simulink library "induction_machine"  (R2025b)
settings: Solver=VariableStepAuto  StartTime=0.0  StopTime=10.0  RelTol=1e-3
undefined symbols (not defined in the file): cp, Jm_model, Lm, Lr, Ls, Rr, Rs
libraries: nesl_utility x41, fl_lib x1, im_uvw_2_lib x1
settings Model: Creator=dbagn  LastModifiedBy=ltnbda

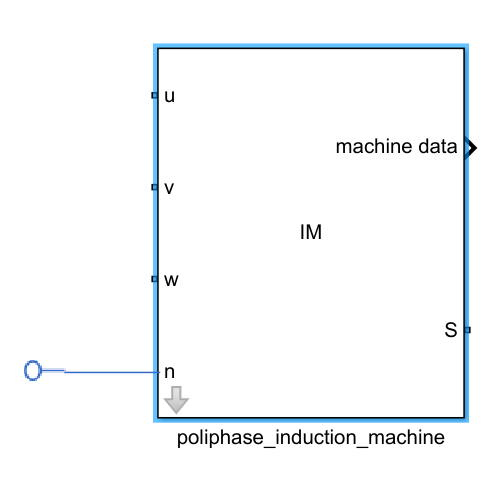
[thumbnail: Simulink's stored preview of the top-level diagram]
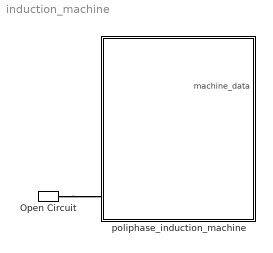
== system induction_machine ==
  Open Circuit : fl_lib/Electrical/Electrical Elements/Open Circuit  v_specify=off  v_priority=None  v=0 V  v_nominal_specify=off  v_nominal_value=1  v_nominal_unit=V
  poliphase_induction_machine : Subsystem  mask{Rs_m=Rs, Ls_m=Ls, Lm_m=Lm, Lr_m=Lr, Rr_m=Rr, Jm_m=Jm_model, bm_m=Tn/omega_m_nom/3, cp_m=cp}
      mask prompts: Rs_m "Stator resistance - Rs [Ohm]"; Ls_m "Stator inductance - Ls [H]"; Lm_m "Mutual inductance - Lm [H]"; Lr_m "Rotor inductance - Lr [H]"; Rr_m "Rotor resistance - Rr [Ohm]"; Jm_m "Load inertia - Jm [kgm^2]"; bm_m "Loadviscosity - bm [Nm*s/rad]"; cp_m "Number of pole pairs"
      mask Display:
      | disp('IM');
      | port_label('lconn', 1, 'u');
      | port_label('lconn', 2, 'v');
      | port_label('lconn', 3, 'w');
      | port_label('lconn', 4, 'n');
      | port_label('output', 1, 'machine data');
      | port_label('rconn',1, 'S');
  connections:
  Open Circuit/LConn1 -- poliphase_induction_machine/LConn4

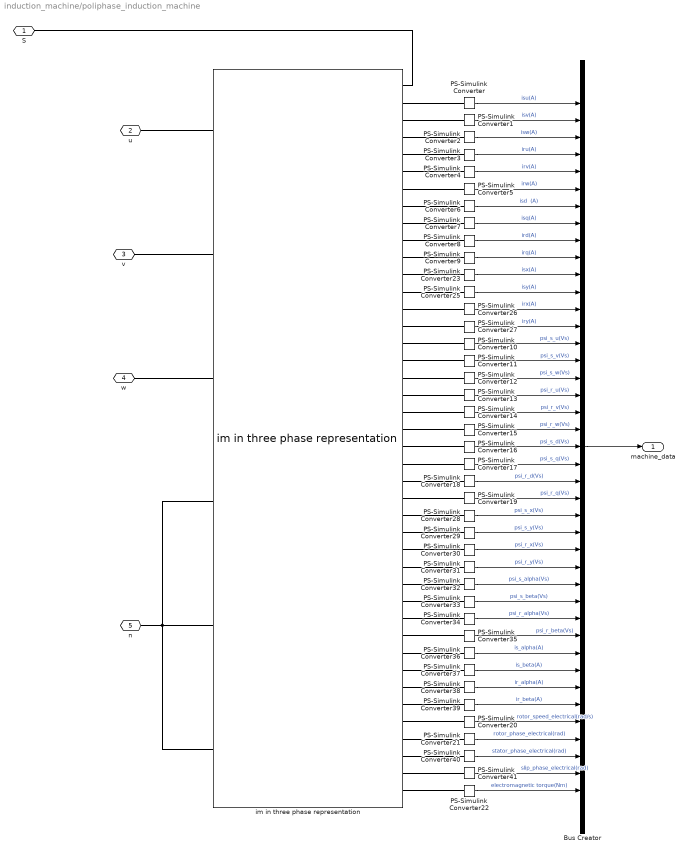
== system induction_machine/poliphase_induction_machine ==
  Bus Creator : BusCreator  Inputs=41
  PS-Simulink Converter{,1..9,23,25..27,36..39} (18 alike) : nesl_utility/PS-Simulink Converter  PhysicalDomain=network_engine_domain  SubClassName=ps_output  LeftPortType=input  RightPortType=output  PseudoPeriodic=off  Frequencies=[]  VectorFormat=1-D array  Unit=A  AffineConversion=off
  PS-Simulink Converter{10..19,28..35} (18 alike) : nesl_utility/PS-Simulink Converter  PhysicalDomain=network_engine_domain  SubClassName=ps_output  LeftPortType=input  RightPortType=output  PseudoPeriodic=off  Frequencies=[]  VectorFormat=1-D array  Unit=V*s  AffineConversion=off
  PS-Simulink Converter20 : nesl_utility/PS-Simulink Converter  PhysicalDomain=network_engine_domain  SubClassName=ps_output  LeftPortType=input  RightPortType=output  PseudoPeriodic=off  Frequencies=[]  VectorFormat=1-D array  Unit=rad/s  AffineConversion=off
  PS-Simulink Converter21 : nesl_utility/PS-Simulink Converter  PhysicalDomain=network_engine_domain  SubClassName=ps_output  LeftPortType=input  RightPortType=output  PseudoPeriodic=off  Frequencies=[]  VectorFormat=1-D array  Unit=rad  AffineConversion=off
  PS-Simulink Converter22 : nesl_utility/PS-Simulink Converter  PhysicalDomain=network_engine_domain  SubClassName=ps_output  LeftPortType=input  RightPortType=output  PseudoPeriodic=off  Frequencies=[]  VectorFormat=1-D array  Unit=N*m  AffineConversion=off
  PS-Simulink Converter40 : nesl_utility/PS-Simulink Converter  PhysicalDomain=network_engine_domain  SubClassName=ps_output  LeftPortType=input  RightPortType=output  PseudoPeriodic=off  Frequencies=[]  VectorFormat=1-D array  Unit=rad  AffineConversion=off
  PS-Simulink Converter41 : nesl_utility/PS-Simulink Converter  PhysicalDomain=network_engine_domain  SubClassName=ps_output  LeftPortType=input  RightPortType=output  PseudoPeriodic=off  Frequencies=[]  VectorFormat=1-D array  Unit=rad  AffineConversion=off
  im in three phase representation : im_uvw_2_lib/im in three phase representation  Lm=Lm_m H  Rs=Rs_m Ohm  Lr=Lr_m H  Ls=Ls_m H  Rr=Rr_m Ohm  Jm=Jm_m kg*m^2  bm=bm_m N*m*s/rad  pp=cp_m  omega_m_specify=off  omega_m_priority=None  omega_m=0 rad/s  omega_m_nominal_specify=off  omega_m_nominal_value=1  omega_m_nominal_unit=rad/s  isu_specify=off  isu_priority=None  isu=0 A  isu_nominal_specify=off  isu_nominal_value=1  isu_nominal_unit=A  isv_specify=off  isv_priority=None  isv=0 A  isv_nominal_specify=off  isv_nominal_value=1  isv_nominal_unit=A  isw_specify=off  isw_priority=None  isw=0 A  isw_nominal_specify=off  isw_nominal_value=1  isw_nominal_unit=A  iru_specify=off  iru_priority=None  iru=0 A  iru_nominal_specify=off  iru_nominal_value=1  iru_nominal_unit=A  irv_specify=off  irv_priority=None  irv=0 A  irv_nominal_specify=off  irv_nominal_value=1  irv_nominal_unit=A  irw_specify=off  irw_priority=None  irw=0 A  irw_nominal_specify=off  irw_nominal_value=1  irw_nominal_unit=A  ird_specify=off  ird_priority=None  ird=0 A  ird_nominal_specify=off  ird_nominal_value=1  ird_nominal_unit=A  irq_specify=off  irq_priority=None  irq=0 A  irq_nominal_specify=off  irq_nominal_value=1  irq_nominal_unit=A  isd_specify=off  isd_priority=None  isd=0 A  isd_nominal_specify=off  isd_nominal_value=1  isd_nominal_unit=A  isq_specify=off  isq_priority=None  isq=0 A  isq_nominal_specify=off  isq_nominal_value=1  isq_nominal_unit=A  irx_specify=off  irx_priority=None  irx=0 A  irx_nominal_specify=off  irx_nominal_value=1  irx_nominal_unit=A  iry_specify=off  iry_priority=None  iry=0 A  iry_nominal_specify=off  iry_nominal_value=1  iry_nominal_unit=A  isx_specify=off  isx_priority=None  isx=0 A  isx_nominal_specify=off  isx_nominal_value=1  isx_nominal_unit=A  isy_specify=off  isy_priority=None  isy=0 A  isy_nominal_specify=off  isy_nominal_value=1  isy_nominal_unit=A  uu_specify=off  uu_priority=None  uu=0 V  uu_nominal_specify=off  uu_nominal_value=1  uu_nominal_unit=V  uv_specify=off  uv_priority=None  uv=0 V  uv_nominal_specify=off  uv_nominal_value=1  uv_nominal_unit=V  uw_specify=off  uw_priority=None  uw=0 V  uw_nominal_specify=off  uw_nominal_value=1  uw_nominal_unit=V  psi_s_u_specify=off  psi_s_u_priority=None  psi_s_u=0 V*s  psi_s_u_nominal_specify=off  psi_s_u_nominal_value=1  psi_s_u_nominal_unit=V*s  psi_s_v_specify=off  psi_s_v_priority=None  psi_s_v=0 V*s  psi_s_v_nominal_specify=off  psi_s_v_nominal_value=1  psi_s_v_nominal_unit=V*s  psi_s_w_specify=off  psi_s_w_priority=None  psi_s_w=0 V*s  psi_s_w_nominal_specify=off  psi_s_w_nominal_value=1  psi_s_w_nominal_unit=V*s  psi_r_u_specify=off  psi_r_u_priority=None  psi_r_u=0 V*s  psi_r_u_nominal_specify=off  psi_r_u_nominal_value=1  psi_r_u_nominal_unit=V*s  psi_r_v_specify=off  psi_r_v_priority=None  psi_r_v=0 V*s  psi_r_v_nominal_specify=off  psi_r_v_nominal_value=1  psi_r_v_nominal_unit=V*s  psi_r_w_specify=off  psi_r_w_priority=None  psi_r_w=0 V*s  psi_r_w_nominal_specify=off  psi_r_w_nominal_value=1  psi_r_w_nominal_unit=V*s  psi_r_d_specify=off  psi_r_d_priority=None  psi_r_d=0 V*s  psi_r_d_nominal_specify=off  psi_r_d_nominal_value=1  psi_r_d_nominal_unit=V*s  psi_r_q_specify=off  psi_r_q_priority=None  psi_r_q=0 V*s  psi_r_q_nominal_specify=off  psi_r_q_nominal_value=1  psi_r_q_nominal_unit=V*s  psi_s_d_specify=off  psi_s_d_priority=None  psi_s_d=0 V*s  psi_s_d_nominal_specify=off  psi_s_d_nominal_value=1  psi_s_d_nominal_unit=V*s  psi_s_q_specify=off  psi_s_q_priority=None  psi_s_q=0 V*s  psi_s_q_nominal_specify=off  psi_s_q_nominal_value=1  psi_s_q_nominal_unit=V*s  psi_r_x_specify=off  psi_r_x_priority=None  psi_r_x=0 V*s  psi_r_x_nominal_specify=off  psi_r_x_nominal_value=1  psi_r_x_nominal_unit=V*s  psi_r_y_specify=off  psi_r_y_priority=None  psi_r_y=0 V*s  psi_r_y_nominal_specify=off  psi_r_y_nominal_value=1  psi_r_y_nominal_unit=V*s  psi_s_x_specify=off  psi_s_x_priority=None  psi_s_x=0 V*s  psi_s_x_nominal_specify=off  psi_s_x_nominal_value=1  psi_s_x_nominal_unit=V*s  psi_s_y_specify=off  psi_s_y_priority=None  psi_s_y=0 V*s  psi_s_y_nominal_specify=off  psi_s_y_nominal_value=1  psi_s_y_nominal_unit=V*s  tau_m_specify=off  tau_m_priority=None  tau_m=0 N*m  tau_m_nominal_specify=off  tau_m_nominal_value=1  tau_m_nominal_unit=N*m  tau_l_specify=off  tau_l_priority=None  tau_l=0 N*m  tau_l_nominal_specify=off  tau_l_nominal_value=1  tau_l_nominal_unit=N*m  theta_m_specify=off  theta_m_priority=None  theta_m=0 rad  theta_m_nominal_specify=off  theta_m_nominal_value=1  theta_m_nominal_unit=rad  theta_slip_specify=off  theta_slip_priority=None  theta_slip=0 rad  theta_slip_nominal_specify=off  theta_slip_nominal_value=1  theta_slip_nominal_unit=rad  theta_s_specify=off  theta_s_priority=None  theta_s=0 rad  theta_s_nominal_specify=off  theta_s_nominal_value=1  theta_s_nominal_unit=rad  omega_slip_specify=off  omega_slip_priority=None  omega_slip=0 rad/s  omega_slip_nominal_specify=off  omega_slip_nominal_value=1  omega_slip_nominal_unit=rad/s  omega_s_specify=off  omega_s_priority=None  omega_s=0 rad/s  omega_s_nominal_specify=off  omega_s_nominal_value=1  omega_s_nominal_unit=rad/s
      settings: InternalSimscapePortConfiguration="{\"Bottom\":[],\"Left\":[{\"id\":\"uu_p\",\"label\":\"uu_p\",\"type\":\"foundation.electrical.electrical\"},{\"id\":\"uv_p\",\"label\":\"uv_p\",\"type\":\"foundation.electrical.electrical\"},{\"id\":\"uw_p\",\"label\":\"uw_p\",\"type\":\"foundation.electrical.electrical\"},{\"id\":\"uu_n\",\"label\":\"uu_n\",\"type\":\"foundation.electrical.electrical\"},{\"id\":\"uv_n\",\"label\":\"uv_n\",\"type\":\"foundation.electrical.electrical\"},{\"id\":\"uw_n\",\"label\":\"uw_n\",\"type\":\"foundation.electrical.electrical\"}],\"Right\":[{\"id\":\"S\",\"label\":\"S\",\"type\":\"foundation.mechanical.rotational.rotational\"},{\"id\":\"isu_out\",\"label\":\"isu\",\"type\":\"output\"},{\"id\":\"isv_out\",\"label\":\"isv\",\"type\":\"output\"},{\"id\":\"isw_out\",\"label\":\"isw\",\"type\":\"output\"},{\"id\":\"iru_out\",\"label\":\"iru\",\"type\":\"output\"},{\"id\":\"irv_out\",\"label\":\"irv\",\"type\":\"output\"},{\"id\":\"irw_out\",\"label\":\"irw\",\"type\":\"output\"},{\"id\":\"isd_out\",\"label\":\"isd\",\"type\":\"output\"},{\"id\":\"isq_out\",\"label\":\"isq\",\"type\":\"output\"},{\"id\":\"ird_out\",\"label\":\"ird\",\"type\":\"output\"},{\"id\":\"irq_out\",\"label\":\"irq\",\"type\":\"output\"},{\"id\":\"isx_out\",\"label\":\"isx\",\"type\":\"output\"},{\"id\":\"isy_out\",\"label\":\"isy\",\"type\":\"output\"},{\"id\":\"irx_out\",\"label\":\"irx\",\"type\":\"output\"},{\"id\":\"iry_out\",\"label\":\"iry\",\"type\":\"output\"},{\"id\":\"psi_s_u_out\",\"label\":\"psi_s_u\",\"type\":\"output\"},{\"id\":\"psi_s_v_out\",\"label\":\"psi_s_v\",\"type\":\"output\"},{\"id\":\"psi_s_w_out\",\"label\":\"psi_s_w\",\"type\":\"output\"},{\"id\":\"psi_r_u_out\",\"label\":\"psi_r_u\",\"type\":\"output\"},{\"id\":\"psi_r_v_out\",\"label\":\"psi_r_v\",\"type\":\"output\"},{\"id\":\"psi_r_w_out\",\"label\":\"psi_r_w\",\"type\":\"output\"},{\"id\":\"psi_s_d_out\",\"label\":\"psi_s_d\",\"type\":\"output\"},{\"id\":\"psi_s_q_out\",\"label\":\"psi_s_q\",\"type\":\"output\"},{\"id\":\"psi_r_d_out\",\"label\":\"psi_r_d\",\"type\":\"output\"},{\"id\":\"psi_r_q_out\",\"label\":\"psi_r_q\",\"type\":\"output\"},{\"id\":\"psi_s_x_out\",\"label\":\"psi_s_x\",\"type\":\"output\"},{\"id\":\"psi_s_y_out\",\"label\":\"psi_s_y\",\"type\":\"output\"},{\"id\":\"psi_r_x_out\",\"label\":\"psi_r_x\",\"type\":\"output\"},{\"id\":\"psi_r_y_out\",\"label\":\"psi_r_y\",\"type\":\"output\"},{\"id\":\"psi_s_alpha_out\",\"label\":\"psi_s_alpha\",\"type\":\"output\"},{\"id\":\"psi_s_beta_out\",\"label\":\"psi_s_beta\",\"type\":\"output\"},{\"id\":\"psi_r_alpha_out\",\"label\":\"psi_r_alpha\",\"type\":\"output\"},{\"id\":\"psi_r_beta_out\",\"label\":\"psi_r_beta\",\"type\":\"output\"},{\"id\":\"is_alpha_out\",\"label\":\"is_alpha\",\"type\":\"output\"},{\"id\":\"is_beta_out\",\"label\":\"is_beta\",\"type\":\"output\"},{\"id\":\"ir_alpha_out\",\"label\":\"ir_alpha\",\"type\":\"output\"},{\"id\":\"ir_beta_out\",\"label\":\"ir_beta\",\"type\":\"output\"},{\"id\":\"omega_m_out\",\"label\":\"rotor_speed(electrical)\",\"type\":\"output\"},{\"id\":\"theta_m_out\",\"label\":\"rotor_phase(electrical)\",\"type\":\"output\"},{\"id\":\"theta_s_out\",\"label\":\"stator_phase(electrical)\",\"type\":\"output\"},{\"id\":\"theta_slip_out\",\"label\":\"slip_phase(electrical)\",\"type\":\"output\"},{\"id\":\"tau_m_out\",\"label\":\"electromagnetic torque\",\"type\":\"output\"}],\"Top\":[]}"
  S : PMIOPort  Side=Right
  u : PMIOPort  Port=2  Side=Left
  v : PMIOPort  Port=3  Side=Left
  w : PMIOPort  Port=4  Side=Left
  n : PMIOPort  Port=5  Side=Left
  machine_data : Outport
  wires:
  PS-Simulink Converter7/1 -> Bus Creator/8  "isq(A)"
  PS-Simulink Converter6/1 -> Bus Creator/7  "isd  (A)"
  PS-Simulink Converter17/1 -> Bus Creator/22  "psi_s_q(Vs)"
  PS-Simulink Converter29/1 -> Bus Creator/26  "psi_s_y(Vs)"
  PS-Simulink Converter39/1 -> Bus Creator/36  "ir_beta(A)"
  PS-Simulink Converter1/1 -> Bus Creator/2  "isv(A)"
  PS-Simulink Converter11/1 -> Bus Creator/16  "psi_s_v(Vs)"
  PS-Simulink Converter26/1 -> Bus Creator/13  "irx(A)"
  PS-Simulink Converter4/1 -> Bus Creator/5  "irv(A)"
  PS-Simulink Converter31/1 -> Bus Creator/28  "psi_r_y(Vs)"
  PS-Simulink Converter34/1 -> Bus Creator/31  "psi_r_alpha(Vs)"
  PS-Simulink Converter8/1 -> Bus Creator/9  "ird(A)"
  PS-Simulink Converter5/1 -> Bus Creator/6  "irw(A)"
  PS-Simulink Converter23/1 -> Bus Creator/11  "isx(A)"
  PS-Simulink Converter/1 -> Bus Creator/1  "isu(A)"
  PS-Simulink Converter41/1 -> Bus Creator/40  "slip_phase_electrical(rad)"
  PS-Simulink Converter21/1 -> Bus Creator/38  "rotor_phase_electrical(rad)"
  PS-Simulink Converter14/1 -> Bus Creator/19  "psi_r_v(Vs)"
  PS-Simulink Converter37/1 -> Bus Creator/34  "is_beta(A)"
  PS-Simulink Converter36/1 -> Bus Creator/33  "is_alpha(A)"
  PS-Simulink Converter22/1 -> Bus Creator/41  "electromagnetic torque(Nm)"
  PS-Simulink Converter9/1 -> Bus Creator/10  "irq(A)"
  PS-Simulink Converter20/1 -> Bus Creator/37  "rotor_speed_electrical(rad/s)"
  PS-Simulink Converter38/1 -> Bus Creator/35  "ir_alpha(A)"
  PS-Simulink Converter30/1 -> Bus Creator/27  "psi_r_x(Vs)"
  PS-Simulink Converter16/1 -> Bus Creator/21  "psi_s_d(Vs)"
  PS-Simulink Converter18/1 -> Bus Creator/23  "psi_r_d(Vs)"
  PS-Simulink Converter40/1 -> Bus Creator/39  "stator_phase_electrical(rad)"
  PS-Simulink Converter27/1 -> Bus Creator/14  "iry(A)"
  PS-Simulink Converter28/1 -> Bus Creator/25  "psi_s_x(Vs)"
  PS-Simulink Converter19/1 -> Bus Creator/24  "psi_r_q(Vs)"
  PS-Simulink Converter15/1 -> Bus Creator/20  "psi_r_w(Vs)"
  PS-Simulink Converter3/1 -> Bus Creator/4  "iru(A)"
  PS-Simulink Converter32/1 -> Bus Creator/29  "psi_s_alpha(Vs)"
  PS-Simulink Converter35/1 -> Bus Creator/32  "psi_r_beta(Vs)"
  PS-Simulink Converter33/1 -> Bus Creator/30  "psi_s_beta(Vs)"
  PS-Simulink Converter2/1 -> Bus Creator/3  "isw(A)"
  PS-Simulink Converter10/1 -> Bus Creator/15  "psi_s_u(Vs)"
  Bus Creator/1 -> machine_data/1
  PS-Simulink Converter12/1 -> Bus Creator/17  "psi_s_w(Vs)"
  PS-Simulink Converter25/1 -> Bus Creator/12  "isy(A)"
  PS-Simulink Converter13/1 -> Bus Creator/18  "psi_r_u(Vs)"
  connections:
  im in three phase representation/RConn6 -- PS-Simulink Converter4/LConn1
  im in three phase representation/RConn27 -- PS-Simulink Converter29/LConn1
  im in three phase representation/RConn32 -- PS-Simulink Converter34/LConn1
  im in three phase representation/LConn3 -- w/RConn1
  PS-Simulink Converter13/LConn1 -- im in three phase representation/RConn19
  PS-Simulink Converter41/LConn1 -- im in three phase representation/RConn41
  im in three phase representation/RConn13 -- PS-Simulink Converter25/LConn1
  im in three phase representation/RConn29 -- PS-Simulink Converter31/LConn1
  im in three phase representation/RConn36 -- PS-Simulink Converter38/LConn1
  im in three phase representation/RConn9 -- PS-Simulink Converter7/LConn1
  im in three phase representation/RConn40 -- PS-Simulink Converter40/LConn1
  PS-Simulink Converter27/LConn1 -- im in three phase representation/RConn15
  PS-Simulink Converter1/LConn1 -- im in three phase representation/RConn3
  PS-Simulink Converter26/LConn1 -- im in three phase representation/RConn14
  im in three phase representation/RConn12 -- PS-Simulink Converter23/LConn1
  im in three phase representation/RConn28 -- PS-Simulink Converter30/LConn1
  PS-Simulink Converter16/LConn1 -- im in three phase representation/RConn22
  im in three phase representation/RConn5 -- PS-Simulink Converter3/LConn1
  PS-Simulink Converter12/LConn1 -- im in three phase representation/RConn18
  im in three phase representation/RConn31 -- PS-Simulink Converter33/LConn1
  im in three phase representation/RConn8 -- PS-Simulink Converter6/LConn1
  im in three phase representation/RConn4 -- PS-Simulink Converter2/LConn1
  im in three phase representation/RConn37 -- PS-Simulink Converter39/LConn1
  PS-Simulink Converter10/LConn1 -- im in three phase representation/RConn16
  im in three phase representation/RConn24 -- PS-Simulink Converter18/LConn1
  PS-Simulink Converter22/LConn1 -- im in three phase representation/RConn42
  PS-Simulink Converter17/LConn1 -- im in three phase representation/RConn23
  im in three phase representation/RConn11 -- PS-Simulink Converter9/LConn1
  PS-Simulink Converter11/LConn1 -- im in three phase representation/RConn17
  im in three phase representation/RConn39 -- PS-Simulink Converter21/LConn1
  im in three phase representation/RConn34 -- PS-Simulink Converter36/LConn1
  PS-Simulink Converter35/LConn1 -- im in three phase representation/RConn33
  im in three phase representation/LConn1 -- u/RConn1
  im in three phase representation/RConn26 -- PS-Simulink Converter28/LConn1
  PS-Simulink Converter14/LConn1 -- im in three phase representation/RConn20
  PS-Simulink Converter19/LConn1 -- im in three phase representation/RConn25
  im in three phase representation/LConn5 -- im in three phase representation/LConn4 -- im in three phase representation/LConn6 -- n/RConn1
  im in three phase representation/RConn30 -- PS-Simulink Converter32/LConn1
  im in three phase representation/RConn10 -- PS-Simulink Converter8/LConn1
  im in three phase representation/RConn35 -- PS-Simulink Converter37/LConn1
  PS-Simulink Converter/LConn1 -- im in three phase representation/RConn2
  PS-Simulink Converter20/LConn1 -- im in three phase representation/RConn38
  im in three phase representation/LConn2 -- v/RConn1
  PS-Simulink Converter5/LConn1 -- im in three phase representation/RConn7
  PS-Simulink Converter15/LConn1 -- im in three phase representation/RConn21
  S/RConn1 -- im in three phase representation/RConn1
